simulink model "schematic"  (R2014b)
settings: Solver=ode45  StartTime=0.0  StopTime=10.0  RelTol=1e-3
settings Model: Creator=danielpihlquist  LastModifiedBy=danielpihlquist
settings DebuggingCC: SignalLabelMismatchMsg=warning  SFcnCompatibilityMsg=warning  StrictBusMsg=WarnOnBusTreatedAsVector  NonBusSignalsTreatedAsBus=warning

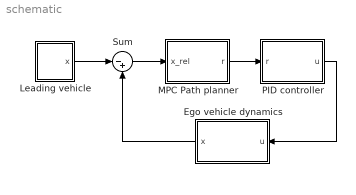
== system schematic ==
  Ego vehicle dynamics : Subsystem
  Leading vehicle : Subsystem
  MPC Path planner : Subsystem
  PID controller : Subsystem
  Sum : Sum  Inputs=|-+
  wires:
  Leading vehicle/1(x) -> Sum/1
  Sum/1 -> MPC Path planner/1(x_rel)
  MPC Path planner/1(r) -> PID controller/1(r)
  PID controller/1(u) -> Ego vehicle dynamics/1(u)
  Ego vehicle dynamics/1(x) -> Sum/2

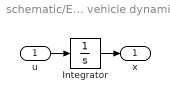
== system schematic/Ego vehicle dynamics ==
  u : Inport
  Integrator : Integrator
  x : Outport
  wires:
  u/1 -> Integrator/1
  Integrator/1 -> x/1

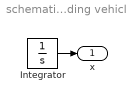
== system schematic/Leading vehicle ==
  Integrator : Integrator
  x : Outport
  wires:
  Integrator/1 -> x/1

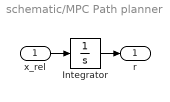
== system schematic/MPC Path planner ==
  x_rel : Inport
  Integrator : Integrator
  r : Outport
  wires:
  x_rel/1 -> Integrator/1
  Integrator/1 -> r/1

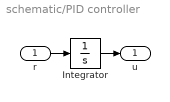
== system schematic/PID controller ==
  r : Inport
  Integrator : Integrator
  u : Outport
  wires:
  Integrator/1 -> u/1
  r/1 -> Integrator/1
